simulink model "PSO_p53_mdm2_simulation"  (R2024a)
settings: Solver=ode15s  StartTime=0.0  StopTime=60  MaxStep=0.1  RelTol=1e-8  AbsTol=1e-8
model workspace (MAT data in the model file):
  x = Simulink.Parameter
  x.Complexity = 'real'
  x.Dimensions = [0 0]
  x.DataType = 'auto'
values from neighbouring files (symbols this model uses):
  dx = positions(i, 5)    [PSO_5_params.m]    (also in PSO_6_params.m; p53_mdm2_simulation.m = 1; params.m = 1; plot_theoretical_pso_params.m = gBest(5))
  dy = positions(i, 6)    [PSO_6_params.m]    (also in p53_mdm2_simulation.m = 1; params.m = 1; plot_theoretical_pso_params.m = gBest(6))
  k1 = positions(i, 1)    [PSO.m]    (also in PSO_3_params.m; PSO_4_params.m; PSO_5_params.m; PSO_6_params.m)
  K1 = 0.1    [p53_mdm2_simulation.m]    (also in params.m)
  k2 = positions(i, 2)    [PSO.m]    (also in PSO_3_params.m; PSO_4_params.m; PSO_5_params.m; PSO_6_params.m)
  K2 = 1    [p53_mdm2_simulation.m]    (also in params.m)
  ks = 2    [p53_mdm2_simulation.m]    (also in params.m)
  n = positions(i,4)    [PSO_4_params.m]    (also in PSO_5_params.m = positions(i, 4); PSO_6_params.m = positions(i, 4); p53_mdm2_simulation.m = 2; params.m = 2)
  tau = positions(i, 3)    [PSO.m]    (also in PSO_3_params.m; PSO_4_params.m; PSO_5_params.m; PSO_6_params.m)
settings Model: Creator=shirley  LastModifiedBy=shirley

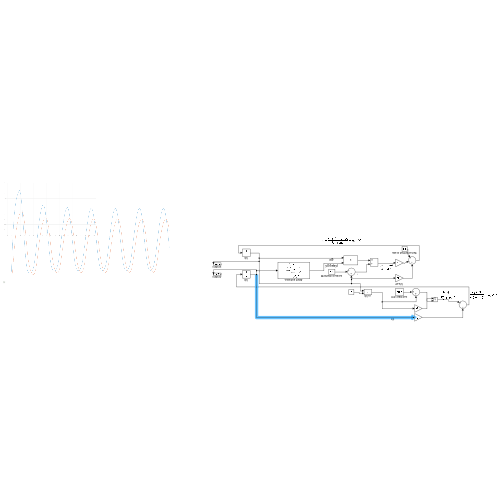
[thumbnail: Simulink's stored preview of the top-level diagram]
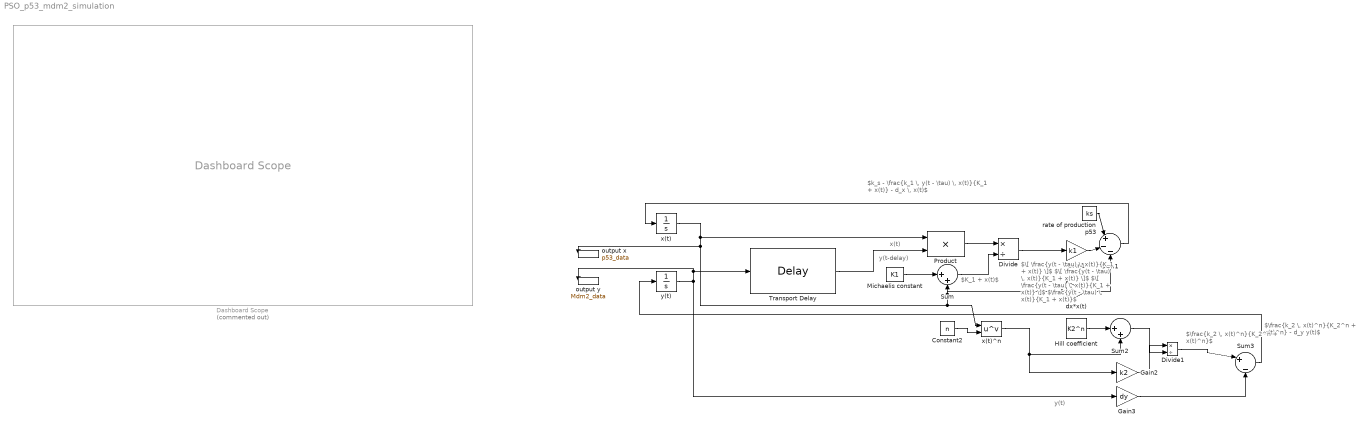
== system PSO_p53_mdm2_simulation ==
  note: y(t)
  note: $K_1 + x(t)$
  note: $\frac{k_2 \, x(t)^n}{K_2^n + x(t)^n} - d_y y(t)$
  note: $k_s - \frac{k_1 \, y(t - \tau) \, x(t)}{K_1 + x(t)} - d_x \, x(t)$
  note: $\frac{k_2 \, x(t)^n}{K_2^n + x(t)^n}$
  note: $\[ \frac{y(t - \tau) \, x(t)}{K_1 + x(t)} \]$ $\[ \frac{y(t - \tau) \, x(t)}{K_1 + x(t)} \]$ $\[ \frac{y(t - \tau) \, x(t)}{K_1 + x(t)} \]$ $\frac{y(t - \tau) \, x(t)}{K_1 + x(t)}$
  note: x(t)
  note: y(t-delay)
  Constant2 : Constant  Value=n
  Dashboard Scope : DashboardScope  Commented=on
  Divide : Product  Inputs=*/
  Divide1 : Product  Inputs=*/
  Gain1 : Gain  Gain=k1
  Gain2 : Gain  Gain=k2
  Gain3 : Gain  Gain=dy
  Hill coefficient : Constant  Value=K2^n
  Michaelis constant : Constant  Value=K1
  Product : Product
  Sum : Sum  Inputs=|++
  Sum1 : Sum  Inputs=|+|-|-
  Sum2 : Sum  Inputs=|++
  Sum3 : Sum  Inputs=|+|-
  Transport Delay : TransportDelay  DelayTime=tau
  dx*x(t) : Gain  Gain=dx
  output x : ToWorkspace  VariableName=p53_data  SampleTime=-1
  output y : ToWorkspace  VariableName=Mdm2_data  SampleTime=-1
  rate of production p53 : Constant  Value=ks
  x(t) : Integrator  InitialCondition=0.2  ContinuousStateAttributes="\"x\""
  x(t)^n : Math  Operator=pow
  y(t) : Integrator  InitialCondition=0.1  ContinuousStateAttributes="\"y\""
  wires:
  Sum1/1 -> x(t)/1
  Divide1/1 -> Sum3/1
  Gain1/1 -> Sum1/2
  rate of production p53/1 -> Sum1/1
  Sum2/1 -> Divide1/2
  Gain2/1 -> Divide1/1
  dx*x(t)/1 -> Sum1/3
  x(t)^n/1 -> Sum2/2, Gain2/1
  Sum3/1 -> y(t)/1
  x(t)/1 -> dx*x(t)/1, Sum/2, x(t)^n/1, output x/1, Product/1
  Hill coefficient/1 -> Sum2/1
  Sum/1 -> Divide/2
  Product/1 -> Divide/1
  Transport Delay/1 -> Product/2
  Divide/1 -> Gain1/1
  y(t)/1 -> Transport Delay/1, output y/1, Gain3/1
  Gain3/1 -> Sum3/2
  Constant2/1 -> x(t)^n/2
  Michaelis constant/1 -> Sum/1
